simulink model "task8_nonlin_model_simu"  (R2017b)
settings: Solver=VariableStepAuto  StartTime=0.0  StopTime=10.0  RelTol=1e-3
values from neighbouring files (symbols this model uses):
  alpha = [alpha1; alpha2]    [OAC_LA_Ass2.m]    (also in testfile.m)
  beta = [beta1; beta2]    [OAC_LA_Ass2.m]    (also in testfile.m)
  gamma = [gamma1; gamma2]    [OAC_LA_Ass2.m]    (also in testfile.m)
  h = evalin('base','h')    [MPC_function.m]    (also in MPC_softcon_function.m; OAC_LA_Ass2.m = [h01; h02]; testfile.m = [h01; h02])
  k = [k1; k2]    [OAC_LA_Ass2.m]    (also in testfile.m)
  x0 = x_eq    [OAC_LA_Ass2.m]    (also in testfile.m = [xe(1); xe(2)])
settings Model: Creator=miko2  LastModifiedBy=lukastotschnig

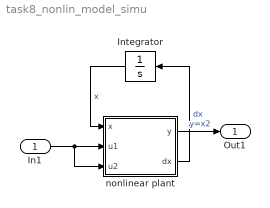
== system task8_nonlin_model_simu ==
  In1 : Inport
  Integrator : Integrator  InitialCondition=x0
  nonlinear plant : MATLAB Function  TreatAsAtomicUnit=on
  Out1 : Outport
  wires:
  nonlinear plant/2(dx) -> Integrator/1  "dx"
  Integrator/1 -> nonlinear plant/1(x)  "x"
  nonlinear plant/1(y) -> Out1/1  "y=x2"
  In1/1 -> nonlinear plant/3(u2), nonlinear plant/2(u1)

== matlab function task8_nonlin_model_simu/nonlinear plant ==
  data: x input; u1 input; u2 input; y output; dx output; k parameter; alpha parameter; beta parameter; gamma parameter; h parameter
function [y, dx]= fcn(x,u1,u2,k,alpha, beta, gamma,h)
    
    % calculate input quantity
    if (beta(1)+gamma(1)*u1) <= 0
        zp1 = 0;
    else
        zp1 = alpha(1) + sqrt( beta(1)+gamma(1)*u1 );
    end
    
    if (beta(2)+gamma(2)*u2) <= 0
        zp2 = 0;
    else
        zp2 = alpha(2) + sqrt( beta(2)+gamma(2)*u2 );
    end
    
   % nonlinear plant description
   dx1 = -k(1)*sqrt(x(1)) + zp1;
   dx2 = -k(2)*sqrt(x(2)) + k(1)*sqrt(x(1))+zp2;
   
   dx = [dx1; dx2];
   y = x(2)-h(2);

end
